simulink model "mortho_bpsk_2u"  (Simulink 6.0)
settings: Solver=ode45  StartTime=0.0  StopTime=0.125 - (1/19200)  RelTol=1e-3
libraries: mspread x6, commsink2 x4, commfilt2 x4, commchan2 x3, commrandsrc2 x2, commseqgen2 x2
CloseFcn:
  | clear spreadSigsOut
settings Model: Creator=akansal  LastModifiedBy=mmclerno  ProdHWDeviceType=Specified
settings DataIOCC: SaveTime=off  SignalLoggingName=spreadSigsOut
settings OptimizationCC: BooleanDataType=off  InlineParams=on  MultiInstanced=off
settings FormatCC: IgnoreBidirectionalLines=off
settings HardwareCC: ProdHWDeviceType=Specified
settings CodeAppCC: SimulinkBlockComments=off
settings GRTTargetCC: TargetFcnLib=iso_c_tmw.mat

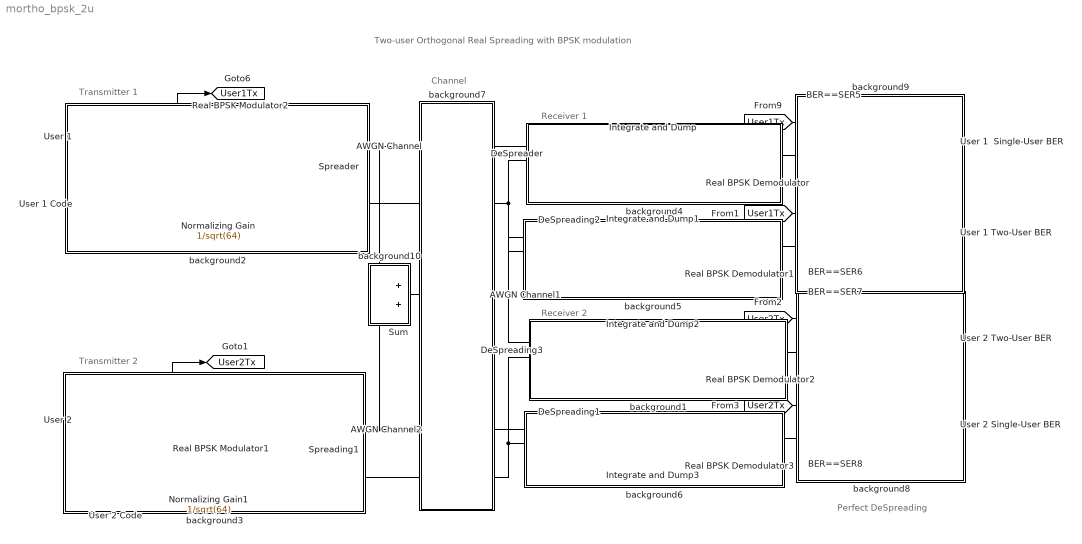
== system mortho_bpsk_2u ==
  note: Two-user Orthogonal Real Spreading with BPSK modulation
  note: Perfect DeSpreading
  note: Transmitter 2
  note: Receiver 1
  note: Channel
  note: Transmitter 1
  note: Receiver 2
  AWGN Channel : commchan2/AWGN Channel  seed=1237  noiseMode="Signal to noise ratio  (SNR)"  EbNodB=10  EsNodB=25  SNRdB=5  bitsPerSym=1  Ps=1  Tsym=ts  variance=1
  AWGN Channel1 : commchan2/AWGN Channel  seed=1237  noiseMode="Signal to noise ratio  (SNR)"  EbNodB=10  EsNodB=25  SNRdB=5  bitsPerSym=1  Ps=1  Tsym=ts  variance=1
  AWGN Channel2 : commchan2/AWGN Channel  seed=1237  noiseMode="Signal to noise ratio  (SNR)"  EbNodB=10  EsNodB=25  SNRdB=5  bitsPerSym=1  Ps=1  Tsym=ts  variance=1
  BER==SER{5..8} (4 alike) : commsink2/Error Rate Calculation  N=0  st_delay=0  cp_mode=Entire frame  subframe=[]  PMode=Port  WsName=ErrorVec  RsMode2=off  stop=off  numErr=100  maxBits=1e6
  DeSpreader : Product  SaturateOnIntegerOverflow=on  InputSameDT=on
  DeSpreading1 : Product  SaturateOnIntegerOverflow=on  InputSameDT=on
  DeSpreading2 : Product  SaturateOnIntegerOverflow=on  InputSameDT=on
  DeSpreading3 : Product  SaturateOnIntegerOverflow=on  InputSameDT=on
  Integrate and Dump{,1..3} (4 alike) : commfilt2/Integrate and Dump  obssamples=64  offsetsamples=0  nodump=off
  Normalizing Gain : Gain  Gain=1/sqrt(64)  SaturateOnIntegerOverflow=on
  Normalizing Gain1 : Gain  Gain=1/sqrt(64)  SaturateOnIntegerOverflow=on
  Real BPSK Demodulator{,1..3} (4 alike) : mspread/Real BPSK Demodulator
  Real BPSK Modulator1 : mspread/Real BPSK Modulator
  Real BPSK Modulator2 : mspread/Real BPSK Modulator
  Spreader : Product  SaturateOnIntegerOverflow=on  InputSameDT=on
  Spreading1 : Product  SaturateOnIntegerOverflow=on  InputSameDT=on
  Sum : Sum  SaturateOnIntegerOverflow=on
  User 1 : commrandsrc2/Random Integer Generator  mul=2  seed=37  Ts=1/19200  frameBased=on  sampPerFrame=1  orient=off
  "User 1 Two-User BER " : Display
  User 1  Single-User BER : Display
  "User 1 Code " : commseqgen2/Hadamard Code Generator  length=64  index=60  ts=1/(19200*64)  frameBased=on  sampPerFrame=64
  User 2 : commrandsrc2/Random Integer Generator  mul=2  seed=631  Ts=1/19200  frameBased=on  sampPerFrame=1  orient=off
  "User 2 Single-User BER " : Display
  User 2 Two-User BER : Display
  User 2 Code : commseqgen2/Hadamard Code Generator  length=64  index=30  ts=1/(19200*64)  frameBased=on  sampPerFrame=64
  background1 : Subsystem
      mask Display: disp('')
  background10 : Subsystem  Orientation=up
      mask Display: disp('')
  background2 : Subsystem
      mask Display: disp('')
  background3 : Subsystem
      mask Display: disp('')
  background4 : Subsystem
      mask Display: disp('')
  background5 : Subsystem
      mask Display: disp('')
  background6 : Subsystem
      mask Display: disp('')
  background7 : Subsystem  Orientation=up
      mask Display: disp('')
  background8 : Subsystem
      mask Display: disp('')
  background9 : Subsystem
      mask Display: disp('')
  tag scope: User1Tx=global, User2Tx=global
  wires:
  "User 1 Code "/1 -> Normalizing Gain/1
  Real BPSK Modulator2/1 -> Spreader/1
  Spreader/1 -> AWGN Channel/1, Sum/1
  AWGN Channel/1 -> DeSpreader/1
  DeSpreader/1 -> Integrate and Dump/1
  Integrate and Dump/1 -> Real BPSK Demodulator/1
  User 2/1 -> [User2Tx], Real BPSK Modulator1/1
  User 2 Code/1 -> Normalizing Gain1/1
  Real BPSK Modulator1/1 -> Spreading1/1
  Normalizing Gain1/1 -> Spreading1/2, DeSpreading3/2, DeSpreading1/2
  Spreading1/1 -> Sum/2, AWGN Channel2/1
  AWGN Channel2/1 -> DeSpreading1/1
  DeSpreading1/1 -> Integrate and Dump3/1
  Sum/1 -> AWGN Channel1/1
  DeSpreading2/1 -> Integrate and Dump1/1
  DeSpreading3/1 -> Integrate and Dump2/1
  AWGN Channel1/1 -> DeSpreading2/1, DeSpreading3/1
  User 1/1 -> [User1Tx], Real BPSK Modulator2/1
  Normalizing Gain/1 -> Spreader/2, DeSpreader/2, DeSpreading2/2
  Real BPSK Demodulator3/1 -> BER==SER8/2
  Real BPSK Demodulator2/1 -> BER==SER7/2
  Real BPSK Demodulator1/1 -> BER==SER6/2
  Integrate and Dump1/1 -> Real BPSK Demodulator1/1
  Integrate and Dump2/1 -> Real BPSK Demodulator2/1
  Integrate and Dump3/1 -> Real BPSK Demodulator3/1
  Real BPSK Demodulator/1 -> BER==SER5/2
  [User1Tx] -> BER==SER5/1
  BER==SER5/1 -> User 1  Single-User BER/1
  [User1Tx] -> BER==SER6/1
  [User2Tx] -> BER==SER7/1
  [User2Tx] -> BER==SER8/1
  BER==SER6/1 -> "User 1 Two-User BER "/1
  BER==SER7/1 -> User 2 Two-User BER/1
  BER==SER8/1 -> "User 2 Single-User BER "/1

== system mortho_bpsk_2u/background1 ==

== system mortho_bpsk_2u/background10 ==

== system mortho_bpsk_2u/background2 ==

== system mortho_bpsk_2u/background3 ==

== system mortho_bpsk_2u/background4 ==

== system mortho_bpsk_2u/background5 ==

== system mortho_bpsk_2u/background6 ==

== system mortho_bpsk_2u/background7 ==

== system mortho_bpsk_2u/background8 ==

== system mortho_bpsk_2u/background9 ==
